simulink model "PthSet_TrqCalc"  (R2018a)
settings: configuration reference "cs_ert" (kept outside this file)
settings Model: DataDictionary=PthSet_TrqCalc.sldd  Creator=zhoutinglin  LastModifiedBy=zhoutinglin

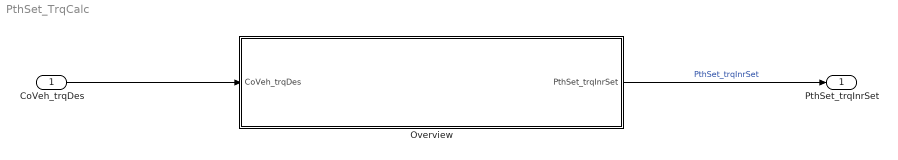
== system PthSet_TrqCalc ==
  CoVeh_trqDes : Inport  Description=Setpoint torque order to the drive train (gearbox output torque)  OutMin=-3000  OutMax=3000  OutDataTypeStr=Torq  Unit=Nm  PortDimensions=[1 1]
  Overview : Subsystem
  PthSet_trqInrSet : Outport
  wires:
  CoVeh_trqDes/1 -> Overview/1(CoVeh_trqDes)
  Overview/1(PthSet_trqInrSet) -> PthSet_trqInrSet/1  "PthSet_trqInrSet"

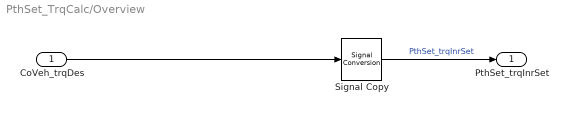
== system PthSet_TrqCalc/Overview ==
  CoVeh_trqDes : Inport  Tag=Nm
  Signal Copy : SignalConversion  OverrideOpt=off
  PthSet_trqInrSet : Outport  Tag=Nm
  wires:
  Signal Copy/1 -> PthSet_trqInrSet/1  "PthSet_trqInrSet"
  CoVeh_trqDes/1 -> Signal Copy/1
